simulink model "fsm_model_test"  (Simulink 8.0)
settings: Solver=ode3  StartTime=0.0  StopTime=inf  FixedStep=0.001  RelTol=1e-3
libraries: simulink x1
settings Model: Creator=caster  LastModifiedBy=caster

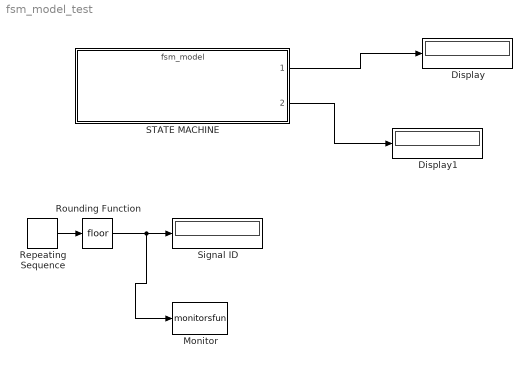
== system fsm_model_test ==
  Display : Display
  Display1 : Display
  Monitor : M-S-Function  FunctionName=monitorsfun
  Repeating Sequence : simulink/Sources/Repeating Sequence  rep_seq_t=0:7  rep_seq_y=[1:8]
  Rounding Function : Rounding
  STATE MACHINE : ModelReference  ModelNameDialog=fsm_model  SimulationMode=Normal  ModelReferenceVersion=1.5  CopyOfModelName=fsm_model  DefaultDataLogging=on
  Signal ID : Display
  wires:
  Rounding Function/1 -> Signal ID/1, Monitor/1
  Repeating Sequence/1 -> Rounding Function/1
  STATE MACHINE/2 -> Display1/1
  STATE MACHINE/1 -> Display/1
